simulink model "Experiment6"  (R2023a)
settings: Solver=VariableStepAuto  StartTime=0.0  StopTime=10.0  RelTol=1e-3
settings Model: Creator=hp 1  LastModifiedBy=hp 1

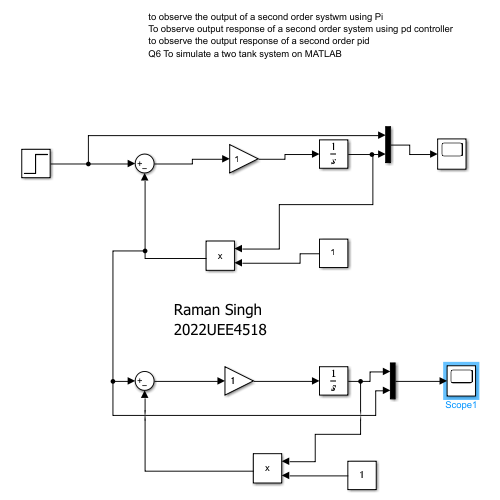
[thumbnail: Simulink's stored preview of the top-level diagram]
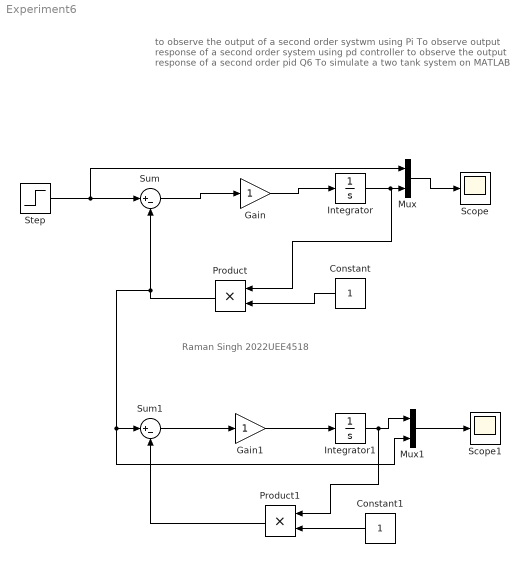
== system Experiment6 ==
  note: Raman Singh
      | 2022UEE4518
  note: to observe the output of a second order systwm using Pi
      | To observe output response of a second order system using pd controller
      | to observe the output response of a second order pid
      | Q6 To simulate a two tank system on MATLAB
  Constant : Constant
  Constant1 : Constant
  Gain : Gain
  Gain1 : Gain
  Integrator : Integrator
  Integrator1 : Integrator
  Mux : Mux  Inputs=2
  Mux1 : Mux  Inputs=2
  Product : Product
  Product1 : Product
  Scope : Scope
  Scope1 : Scope
  Step : Step  SampleTime=0
  Sum : Sum  Inputs=|+-
  Sum1 : Sum  Inputs=|+-
  wires:
  Step/1 -> Mux/1, Sum/1
  Sum/1 -> Gain/1
  Gain/1 -> Integrator/1
  Integrator/1 -> Mux/2, Product/1
  Constant/1 -> Product/2
  Mux/1 -> Scope/1
  Sum1/1 -> Gain1/1
  Gain1/1 -> Integrator1/1
  Integrator1/1 -> Product1/1, Mux1/1
  Product/1 -> Mux1/2, Sum1/1, Sum/2
  Mux1/1 -> Scope1/1
  Product1/1 -> Sum1/2
  Constant1/1 -> Product1/2
